simulink model "VAB_non_linear_Discrete_function"  (R2019b)
settings: Solver=VariableStepAuto  StartTime=0.0  StopTime=t_end  FixedStep=Ts  RelTol=1e-3
values from neighbouring files (symbols this model uses):
  Ts = evalin('base', 'Ts')    [controllore.m]    (also in controllore_motore.m = evalin('base', 'Ts_motore'); phi_p_filter.m; theta_p_filter.m)
undefined symbols (not defined in the file or in its folder): controllore, controllore_motore, m_c_simulazione, motor, phi_iniziale, phi_p_iniziale, phi_p_setpoint, phi_secondo, sensitivity_arduino, theta_iniziale, theta_p_iniziale, theta_secondo, Ts_motore
libraries: simulink x1
settings Model: Creator=miche  LastModifiedBy=AndreaCalegari

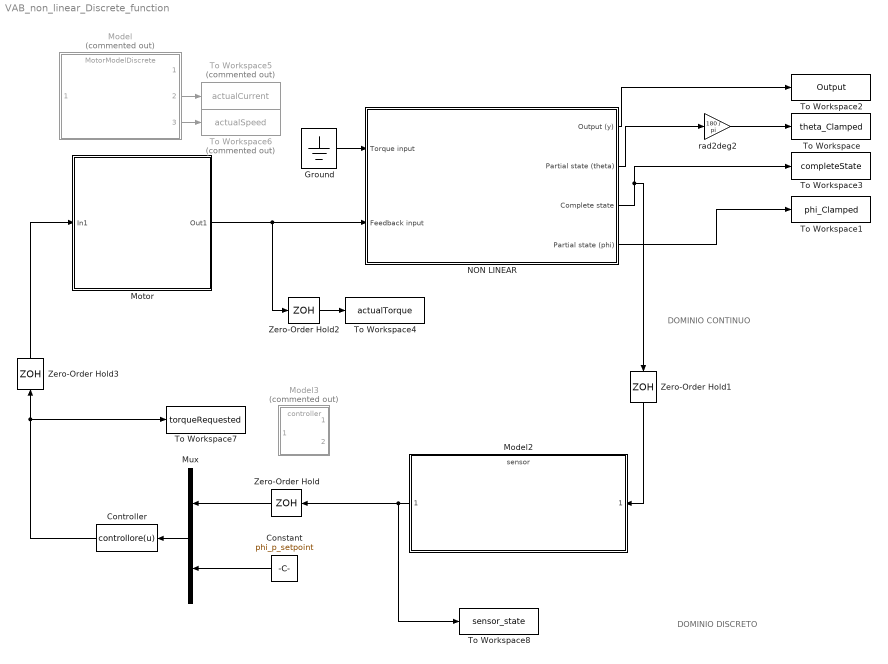
== system VAB_non_linear_Discrete_function ==
  note: DOMINIO DISCRETO
  note: DOMINIO CONTINUO
  Constant : Constant  Value=phi_p_setpoint
  Controller : MATLABFcn  MATLABFcn=controllore(u)
  Ground : Ground
  Model : ModelReference  Commented=on  ModelNameDialog=MotorModelDiscrete.slx  SimulationMode=Normal  ModelReferenceVersion=1.14
  Model2 : ModelReference  ModelNameDialog=sensor.slx  SimulationMode=Normal  ModelReferenceVersion=1.5
  Model3 : ModelReference  Commented=on  ModelNameDialog=controller.slx  SimulationMode=Normal  ModelReferenceVersion=1.18
  Motor : Subsystem
  Mux : Mux  Inputs=2
  NON LINEAR : Subsystem
  To Workspace : ToWorkspace  VariableName=theta_Clamped  SampleTime=-1
  To Workspace1 : ToWorkspace  VariableName=phi_Clamped  SampleTime=-1
  To Workspace2 : ToWorkspace  VariableName=Output  SampleTime=-1
  To Workspace3 : ToWorkspace  VariableName=completeState  SampleTime=-1
  To Workspace4 : ToWorkspace  VariableName=actualTorque  SampleTime=-1
  To Workspace5 : ToWorkspace  Commented=on  VariableName=actualCurrent  SampleTime=-1
  To Workspace6 : ToWorkspace  Commented=on  VariableName=actualSpeed  SampleTime=-1
  To Workspace7 : ToWorkspace  VariableName=torqueRequested  SampleTime=-1
  To Workspace8 : ToWorkspace  VariableName=sensor_state  SampleTime=-1
  Zero-Order Hold{,1..3} (4 alike) : ZeroOrderHold  SampleTime=Ts
  rad2deg2 : Gain  Gain=180 / pi
  wires:
  Model2/1 -> To Workspace8/1, Zero-Order Hold/1
  Constant/1 -> Mux/2
  Zero-Order Hold1/1 -> Model2/1
  Controller/1 -> To Workspace7/1, Zero-Order Hold3/1
  NON LINEAR/1(Output (y)) -> To Workspace2/1
  Zero-Order Hold3/1 -> Motor/1(In1)
  Model/3 -> To Workspace6/1
  NON LINEAR/2(Partial state (theta)) -> rad2deg2/1
  Model/2 -> To Workspace5/1
  rad2deg2/1 -> To Workspace/1
  NON LINEAR/4(Partial state (phi)) -> To Workspace1/1
  NON LINEAR/3("Complete state ") -> To Workspace3/1, Zero-Order Hold1/1
  Motor/1(Out1) -> Zero-Order Hold2/1, NON LINEAR/2(Feedback input)
  Ground/1 -> NON LINEAR/1(Torque input)
  Zero-Order Hold/1 -> Mux/1
  Zero-Order Hold2/1 -> To Workspace4/1
  Mux/1 -> Controller/1

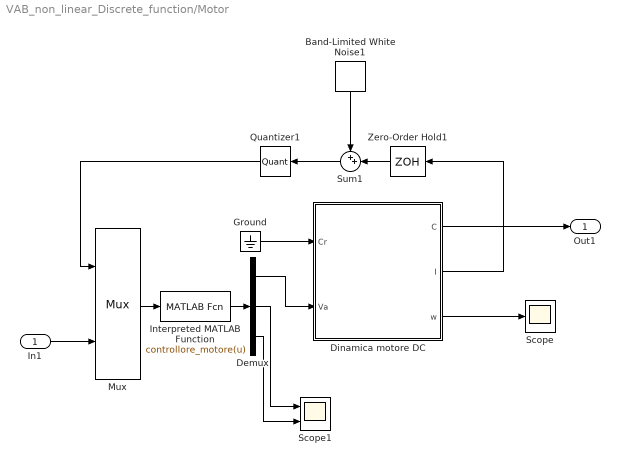
== system VAB_non_linear_Discrete_function/Motor ==
  In1 : Inport  PortDimensions=1
  Band-Limited White Noise1 : simulink/Sources/Band-Limited White Noise  Cov=[0.0001]  Ts=0.001  seed=[23341]
  Demux : Demux  Outputs=3
  Dinamica motore DC : Subsystem
  Ground : Ground
  Interpreted MATLAB Function : MATLABFcn  MATLABFcn=controllore_motore(u)  OutputDimensions=3
  Mux : Mux  Inputs=2
      settings: DisplayOption=signals
  Quantizer1 : Quantizer  QuantizationInterval=1/sensitivity_arduino
  Scope : Scope
  Scope1 : Scope  NumInputPorts=2
  Sum1 : Sum  Inputs=++|
  Zero-Order Hold1 : ZeroOrderHold  SampleTime=Ts_motore
  Out1 : Outport  PortDimensions=1
  wires:
  Dinamica motore DC/1(C) -> Out1/1
  In1/1 -> Mux/2
  Mux/1 -> Interpreted MATLAB Function/1
  Band-Limited White Noise1/1 -> Sum1/1
  Zero-Order Hold1/1 -> Sum1/2
  Dinamica motore DC/2(I) -> Zero-Order Hold1/1
  Sum1/1 -> Quantizer1/1
  Quantizer1/1 -> Mux/1
  Ground/1 -> Dinamica motore DC/1(Cr)
  Dinamica motore DC/3(w) -> Scope/1
  Interpreted MATLAB Function/1 -> Demux/1
  Demux/1 -> Dinamica motore DC/2(Va)
  Demux/2 -> Scope1/1
  Demux/3 -> Scope1/2

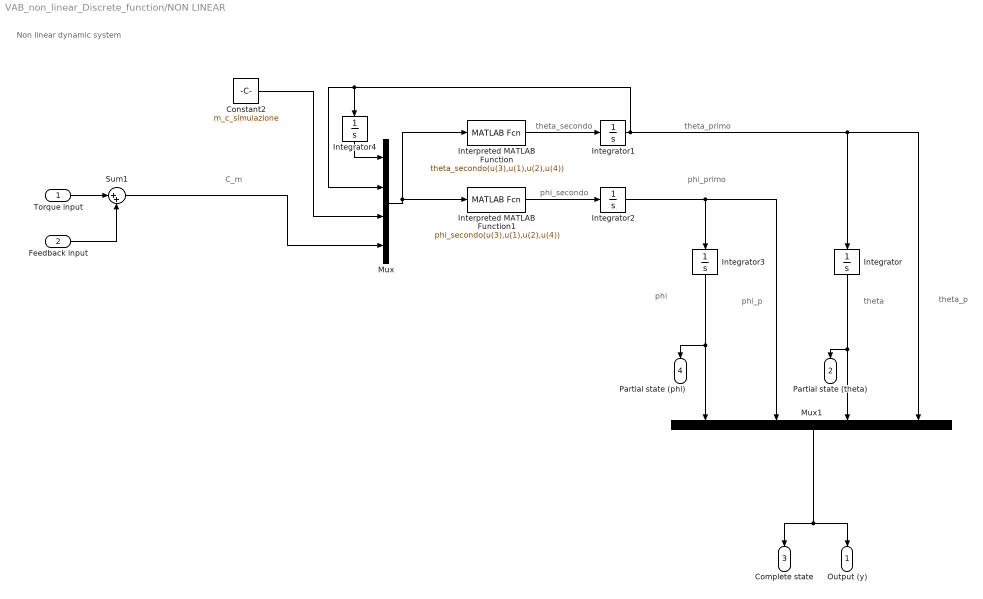
== system VAB_non_linear_Discrete_function/NON LINEAR ==
  note: Non linear dynamic system
  note: phi_primo
  note: phi
  note: theta_p
  note: theta
  note: phi_p
  note: phi_secondo
  note: C_m
  note: theta_secondo
  note: theta_primo
  Torque input : Inport  PortDimensions=1
  Feedback input : Inport  Port=2  PortDimensions=1
  Constant2 : Constant  Value=m_c_simulazione
  Integrator : Integrator  InitialCondition=theta_iniziale
  Integrator1 : Integrator  InitialCondition=theta_p_iniziale  UpperSaturationLimit=100  LowerSaturationLimit=-100
  Integrator2 : Integrator  InitialCondition=phi_p_iniziale
  Integrator3 : Integrator  InitialCondition=phi_iniziale
  Integrator4 : Integrator  InitialCondition=theta_iniziale
  Interpreted MATLAB Function : MATLABFcn  MATLABFcn=theta_secondo(u(3),u(1),u(2),u(4))  OutputDimensions=1
  Interpreted MATLAB Function1 : MATLABFcn  MATLABFcn=phi_secondo(u(3),u(1),u(2),u(4))  OutputDimensions=1
  Mux : Mux
      settings: DisplayOption=signals
  Mux1 : Mux
  Sum1 : Sum  Inputs=|++
  Output (y) : Outport
  Partial state (theta) : Outport  Port=2
  "Complete state " : Outport  Port=3
  Partial state (phi) : Outport  Port=4
  wires:
  Feedback input/1 -> Sum1/2
  Torque input/1 -> Sum1/1
  Integrator3/1 -> Partial state (phi)/1, Mux1/1
  Constant2/1 -> Mux/3
  Sum1/1 -> Mux/4
  Integrator4/1 -> Mux/1
  Interpreted MATLAB Function1/1 -> Integrator2/1
  Integrator2/1 -> Mux1/2, Integrator3/1
  Integrator1/1 -> Integrator4/1, Mux/2, Mux1/4, Integrator/1
  Integrator/1 -> Partial state (theta)/1, Mux1/3
  Interpreted MATLAB Function/1 -> Integrator1/1
  Mux1/1 -> Output (y)/1, "Complete state "/1
  Mux/1 -> Interpreted MATLAB Function/1, Interpreted MATLAB Function1/1

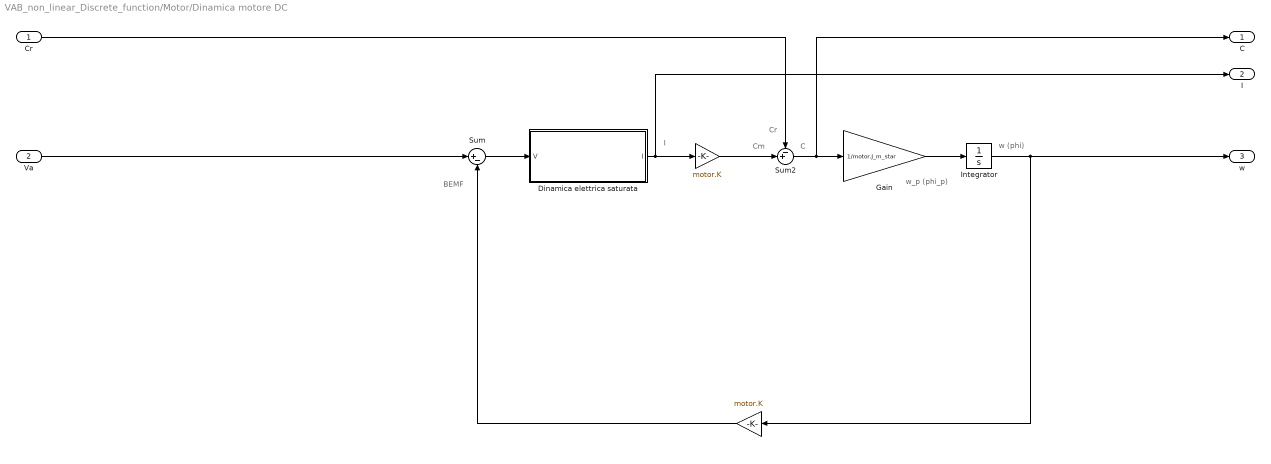
== system VAB_non_linear_Discrete_function/Motor/Dinamica motore DC ==
  note: w (phi)
  note: C
  note: I
  note: Cm
  note: Cr
  note: w_p (phi_p)
  note: BEMF
  Cr : Inport
  Va : Inport  Port=2
  " " : Gain  Gain=motor.K
  " " : Gain  Gain=motor.K
  "Dinamica elettrica saturata " : Subsystem
  Gain : Gain  Gain=1/motor.J_m_star
  Integrator : Integrator
  Sum : Sum  Inputs=|+-
  Sum2 : Sum  Inputs=-+|
  C : Outport
  I : Outport  Port=2  PortDimensions=1
  w : Outport  Port=3
  wires:
  " "/1 -> Sum2/2
  Sum2/1 -> Gain/1, C/1
  Integrator/1 -> " "/1, w/1
  "Dinamica elettrica saturata "/1(I) -> I/1, " "/1
  Cr/1 -> Sum2/1
  " "/1 -> Sum/2
  Va/1 -> Sum/1
  Sum/1 -> "Dinamica elettrica saturata "/1(V)
  Gain/1 -> Integrator/1

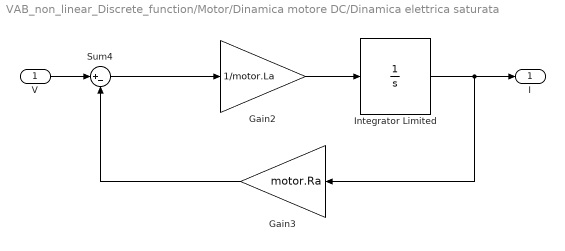
== system VAB_non_linear_Discrete_function/Motor/Dinamica motore DC/Dinamica elettrica saturata  ==
  V : Inport
  Gain2 : Gain  Gain=1/motor.La
  Gain3 : Gain  Gain=motor.Ra
  Integrator Limited : Integrator  LimitOutput=on  UpperSaturationLimit=motor.Imax  LowerSaturationLimit=-motor.Imax
  Sum4 : Sum  Inputs=|+-
  I : Outport
  wires:
  Gain3/1 -> Sum4/2
  Sum4/1 -> Gain2/1
  Gain2/1 -> Integrator Limited/1
  Integrator Limited/1 -> I/1, Gain3/1
  V/1 -> Sum4/1
